simulink model "model"  (R2023b)
settings: Solver=VariableStepAuto  StartTime=0.0  StopTime=10.0  RelTol=1e-3
values from neighbouring files (symbols this model uses):
  f = 50    [model_script.m]    (also in setup_environment.m; test_setup.m)
  L_01_1 = l.*l1.*m_actual    [model_script.m]    (also in setup_environment.m)
  L_01_2 = l.*l1.*(1-m_actual)    [model_script.m]    (also in setup_environment.m)
  L_12 = l.*l2    [model_script.m]    (also in setup_environment.m)
  L_23 = l.*l3    [model_script.m]    (also in setup_environment.m)
  L_S = 16E-3    (= 0.016)    [model_script.m]    (also in setup_environment.m; test_setup.m = 0.01658)
  R_01_1 = r.*l1.*m_actual    [model_script.m]    (also in setup_environment.m)
  R_01_2 = r.*l1.*(1-m_actual)    [model_script.m]    (also in setup_environment.m)
  R_12 = r.*l2    [model_script.m]    (also in setup_environment.m)
  R_23 = r.*l3    [model_script.m]    (also in setup_environment.m)
  R_S = 0.8913    [model_script.m]    (also in setup_environment.m; test_setup.m = 0.8929)
  V_S = 11000    [model_script.m]    (also in setup_environment.m; test_setup.m)
libraries: spsRMSLib x6, spsThreePhaseSeriesRLCBranchLib x4, spsThreePhaseParallelRLCLoadLib x3, spsThreePhaseVIMeasurementLib x1, spsThreePhaseFaultLib x1, spsThreePhaseSourceLib x1, sps_lib x1
settings Model: Creator=CoolBose  LastModifiedBy=CoolBose

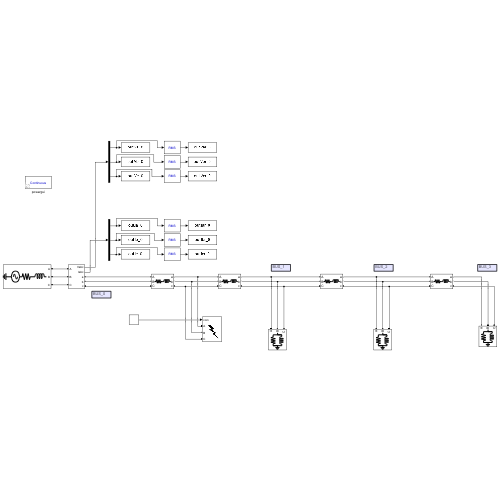
[thumbnail: Simulink's stored preview of the top-level diagram]
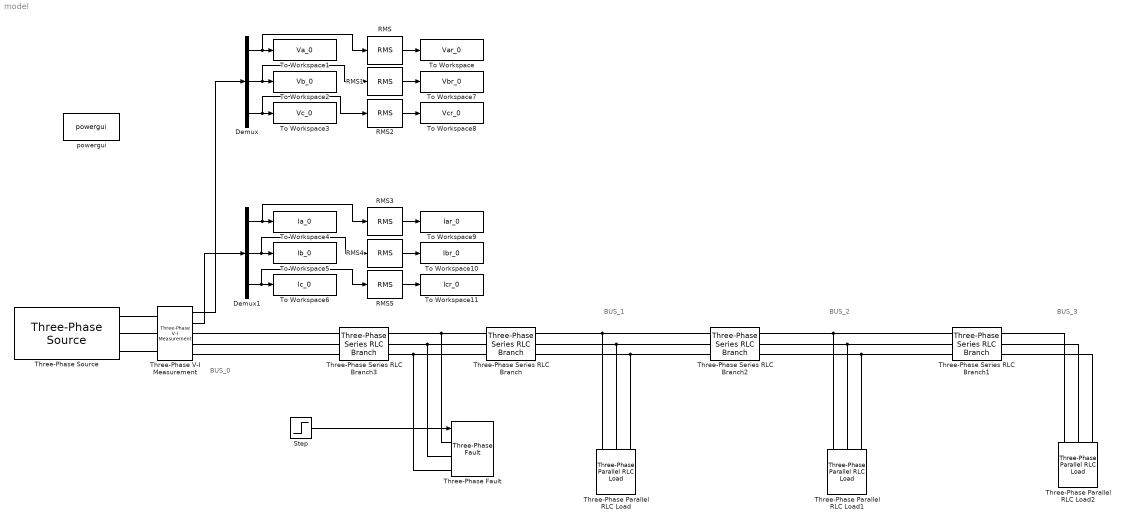
== system model ==
  note: BUS_0
  note: BUS_1
  note: BUS_2
  note: BUS_3
  Demux : Demux  Outputs=3
  Demux1 : Demux  Outputs=3
  RMS{,1..2,4..5} (5 alike) : spsRMSLib/RMS  TrueRMS=off  Freq=f  RMSInit=120  Ts=0
  RMS3 : spsRMSLib/RMS  TrueRMS=off  Freq=60  RMSInit=f  Ts=0
  Step : Step  Time=5  SampleTime=0
  Three-Phase Parallel RLC Load : spsThreePhaseParallelRLCLoadLib/Three-Phase Parallel RLC Load  LConnTagsString=A|B|C  Configuration=Y (grounded)  NominalVoltage=V_L1  Vabc=[1e3 1e3 1e3]  Vabcp=[1e3 1e3 1e3]  NominalFrequency=f  UnbalancedPower=off  ActivePower=P_L1  InductivePower=Q_L1  CapacitivePower=0  Pabc=[10e3 9e3 11e3]  QLabc=[100 90 110]  QCabc=[100 90 110]  Pabcp=[10e3 9e3 11e3]  QLabcp=[100 90 110]  QCabcp=[100 90 110]  Measurements=None  LoadType=constant Z
  Three-Phase Parallel RLC Load1 : spsThreePhaseParallelRLCLoadLib/Three-Phase Parallel RLC Load  LConnTagsString=A|B|C  Configuration=Y (grounded)  NominalVoltage=V_L2  Vabc=[1e3 1e3 1e3]  Vabcp=[1e3 1e3 1e3]  NominalFrequency=f  UnbalancedPower=off  ActivePower=P_L2  InductivePower=Q_L2  CapacitivePower=0  Pabc=[10e3 9e3 11e3]  QLabc=[100 90 110]  QCabc=[100 90 110]  Pabcp=[10e3 9e3 11e3]  QLabcp=[100 90 110]  QCabcp=[100 90 110]  Measurements=None  LoadType=constant Z
  Three-Phase Parallel RLC Load2 : spsThreePhaseParallelRLCLoadLib/Three-Phase Parallel RLC Load  LConnTagsString=A|B|C  Configuration=Y (grounded)  NominalVoltage=V_L3  Vabc=[1e3 1e3 1e3]  Vabcp=[1e3 1e3 1e3]  NominalFrequency=f  UnbalancedPower=off  ActivePower=P_L3  InductivePower=Q_L3  CapacitivePower=0  Pabc=[10e3 9e3 11e3]  QLabc=[100 90 110]  QCabc=[100 90 110]  Pabcp=[10e3 9e3 11e3]  QLabcp=[100 90 110]  QCabcp=[100 90 110]  Measurements=None  LoadType=constant Z
  Three-Phase Series RLC Branch : spsThreePhaseSeriesRLCBranchLib/Three-Phase Series RLC Branch  LConnTagsString=A|B|C  RConnTagsString=A|B|C  BranchType=RL  Resistance=R_01_2  Inductance=L_01_2  Capacitance=1e-6  Measurements=None
  Three-Phase Series RLC Branch1 : spsThreePhaseSeriesRLCBranchLib/Three-Phase Series RLC Branch  LConnTagsString=A|B|C  RConnTagsString=A|B|C  BranchType=RL  Resistance=R_23  Inductance=L_23  Capacitance=1e-6  Measurements=None
  Three-Phase Series RLC Branch2 : spsThreePhaseSeriesRLCBranchLib/Three-Phase Series RLC Branch  LConnTagsString=A|B|C  RConnTagsString=A|B|C  BranchType=RL  Resistance=R_12  Inductance=L_12  Capacitance=1e-6  Measurements=None
  Three-Phase Series RLC Branch3 : spsThreePhaseSeriesRLCBranchLib/Three-Phase Series RLC Branch  LConnTagsString=A|B|C  RConnTagsString=A|B|C  BranchType=RL  Resistance=R_01_1  Inductance=L_01_1  Capacitance=1e-6  Measurements=None
  Three-Phase V-I Measurement : spsThreePhaseVIMeasurementLib/Three-Phase V-I Measurement  VoltageMeasurement=phase-to-ground  SetLabelV=off  LabelV=Vabc  Vpu=off  VpuLL=off  CurrentMeasurement=yes  SetLabelI=off  LabelI=Iabc  Ipu=off  Pbase=100e6  Vbase=500e3  OutputType=Complex  PhasorSimulation=off  PSBequivalent=0
  Three-Phase Fault : spsThreePhaseFaultLib/Three-Phase Fault  InitialStates=0  FaultA=on  FaultB=off  FaultC=off  GroundFault=on  SwitchTimes="[1/60  5/60]"  External=on  SwitchStatus=NaN  FaultResistance=0.001  GroundResistance=0.01  SnubberResistance=1e6  SnubberCapacitance=inf  Measurements=None
  Three-Phase Source : spsThreePhaseSourceLib/Three-Phase Source  InternalConnection=Yg  VoltagePhases=off  Voltage=V_S  PhaseAngle=0  Voltage_phases=[25e3 25e3 25e3]/sqrt(3)  PhaseAngles_phases=[0 -120 +120]  Frequency=f  NonIdealSource=on  SpecifyImpedance=off  Resistance=R_S  Inductance=L_S  ShortCircuitLevel=100e6  BaseVoltage=V_S  XRratio=7  BusType=swing  Pref=10e3  Qref=0  Prefabc=[10e3, 10e3, 10e3]  Qrefabc=[0, 0, 0]  Qmin=-inf  Qmax=inf
  To Workspace : ToWorkspace  VariableName=Var_0  SaveFormat=Timeseries  SampleTime=-1
  To Workspace1 : ToWorkspace  VariableName=Va_0  SampleTime=-1
  To Workspace10 : ToWorkspace  VariableName=Ibr_0  SaveFormat=Timeseries  SampleTime=-1
  To Workspace11 : ToWorkspace  VariableName=Icr_0  SaveFormat=Timeseries  SampleTime=-1
  To Workspace2 : ToWorkspace  VariableName=Vb_0  SampleTime=-1
  To Workspace3 : ToWorkspace  VariableName=Vc_0  SampleTime=-1
  To Workspace4 : ToWorkspace  VariableName=Ia_0  SaveFormat=Structure With Time  SampleTime=-1
  To Workspace5 : ToWorkspace  VariableName=Ib_0  SaveFormat=Structure With Time  SampleTime=-1
  To Workspace6 : ToWorkspace  VariableName=Ic_0  SaveFormat=Structure With Time  SampleTime=-1
  To Workspace7 : ToWorkspace  VariableName=Vbr_0  SaveFormat=Timeseries  SampleTime=-1
  To Workspace8 : ToWorkspace  VariableName=Vcr_0  SaveFormat=Timeseries  SampleTime=-1
  To Workspace9 : ToWorkspace  VariableName=Iar_0  SaveFormat=Timeseries  SampleTime=-1
  powergui : sps_lib/powergui  Priority=1  SimulationMode=Continuous  SampleTime=50e-6  frequency=f  Iterations=50  frequencyindice=50  Pbase=100e6  ErrMax=1e-4  UnitsV=kV  UnitsW=MW  buscounter=0  FunctionMessages=off  echomessages=off  EnableUseOfTLC=off  CurrentSourceSwitches=off  DisableSnubberDevices=off  DisableRonSwitches=off  DisableVfSwitches=off  DisplayEquations=off  AutomaticDiscreteSolvers=off  SolverType=Tustin/Backward Euler (TBE)  Interpol=off  ExternalGateDelay=off  methode=off  Ts=100  x0status=blocks  SPID=on  SwTol=0  HookPort=off  NonlinearTolerance=1e-4  nMaxIteration=100  ContinueOnMaxIteration=off  RestoreLinks=warning  ResistiveCurrentMeasurement=off  Frange=[0:2:500]  Ylog=off  Xlog=on  ShowGrid=off  save=off  variable=ZData  structure=0  ZoomFFT=off  StartTime=0.0  cycles=1  DisplayStyle=1  fundamental=60  FreqAxis=off  MaxFrequency=1000  frequencyindicesteady=1  RmsSteady=1  display=off
  wires:
  Step/1 -> Three-Phase Fault/1
  Three-Phase V-I Measurement/1 -> Demux/1
  Three-Phase V-I Measurement/2 -> Demux1/1
  Demux/1 -> RMS/1, To Workspace1/1
  Demux/2 -> RMS1/1, To Workspace2/1
  Demux/3 -> RMS2/1, To Workspace3/1
  Demux1/2 -> RMS4/1, To Workspace5/1
  Demux1/1 -> RMS3/1, To Workspace4/1
  Demux1/3 -> RMS5/1, To Workspace6/1
  RMS/1 -> To Workspace/1
  RMS1/1 -> To Workspace7/1
  RMS2/1 -> To Workspace8/1
  RMS3/1 -> To Workspace9/1
  RMS4/1 -> To Workspace10/1
  RMS5/1 -> To Workspace11/1
  connections:
  Three-Phase Series RLC Branch/RConn1 -- Three-Phase Parallel RLC Load/LConn1 -- Three-Phase Series RLC Branch2/LConn1
  Three-Phase Series RLC Branch2/LConn2 -- Three-Phase Parallel RLC Load/LConn2 -- Three-Phase Series RLC Branch/RConn2
  Three-Phase Series RLC Branch/RConn3 -- Three-Phase Parallel RLC Load/LConn3 -- Three-Phase Series RLC Branch2/LConn3
  Three-Phase Series RLC Branch2/RConn1 -- Three-Phase Series RLC Branch1/LConn1 -- Three-Phase Parallel RLC Load1/LConn1
  Three-Phase Series RLC Branch2/RConn2 -- Three-Phase Series RLC Branch1/LConn2 -- Three-Phase Parallel RLC Load1/LConn2
  Three-Phase Series RLC Branch2/RConn3 -- Three-Phase Series RLC Branch1/LConn3 -- Three-Phase Parallel RLC Load1/LConn3
  Three-Phase V-I Measurement/LConn3 -- Three-Phase Source/RConn3
  Three-Phase V-I Measurement/LConn2 -- Three-Phase Source/RConn2
  Three-Phase Source/RConn1 -- Three-Phase V-I Measurement/LConn1
  Three-Phase Parallel RLC Load2/LConn1 -- Three-Phase Series RLC Branch1/RConn1
  Three-Phase Series RLC Branch1/RConn2 -- Three-Phase Parallel RLC Load2/LConn2
  Three-Phase Parallel RLC Load2/LConn3 -- Three-Phase Series RLC Branch1/RConn3
  Three-Phase Series RLC Branch3/LConn1 -- Three-Phase V-I Measurement/RConn1
  Three-Phase Series RLC Branch3/LConn2 -- Three-Phase V-I Measurement/RConn2
  Three-Phase Series RLC Branch3/LConn3 -- Three-Phase V-I Measurement/RConn3
  Three-Phase Series RLC Branch3/RConn3 -- Three-Phase Fault/LConn3 -- Three-Phase Series RLC Branch/LConn3
  Three-Phase Series RLC Branch3/RConn2 -- Three-Phase Fault/LConn2 -- Three-Phase Series RLC Branch/LConn2
  Three-Phase Series RLC Branch3/RConn1 -- Three-Phase Fault/LConn1 -- Three-Phase Series RLC Branch/LConn1
